simulink model "GolfSwing"  (R2024b)
settings: Solver=VariableStepAuto  StartTime=0.0  StopTime=StopTime  MaxStep=0.001  RelTol=1e-3
PreLoadFcn:
  | cd(matlabdrive);
  | cd '2DModel';
PostLoadFcn:
  | %run SCRIPT_mdlWksGenerate.m;
  | mdlWks=get_param('GolfSwing','ModelWorkspace');
  | mdlWks.DataSource = 'MAT-File';
  | mdlWks.FileName = 'ModelInputs.mat';
  | mdlWks.reload;
model workspace: external: MAT-File ModelInputs.mat (data not in the file)
undefined symbols (not defined in the file or in its folder): GlobalGain, HipConstant, HipDampening, HipTimeGain, KillDampFinalValue, KillDampInitialValue, KillswitchFinalValue, KillswitchInitialValue, KillswitchStepTime, LElbowConstant, LElbowDampening, LElbowTimeGain, LScapConstant, LScapDampening, LScapPositionGain, LScapTimeGain, LShoulderConstant, LShoulderDampening, LShoulderTimeGain, LWristConstant, LWristDampening, LWristTimeGain, RElbowConstant, RElbowDampening, RElbowTimeGain, RScapConstant, RScapDampening, RScapPositionGain, RScapTimeGain, RShoulderConstant, RShoulderDampening, RShoulderTimeGain, RWristConstant, RWristDampening, RWristTimeGain, TorsoConstant, TorsoDampening, TorsoPositionGain, TorsoTimeGain, WristGain, X, Y, Z
libraries: nesl_utility x207, sm_lib x106, matrix_library x11, simulink_extras x2, simulink x1
(part 4 of 6)

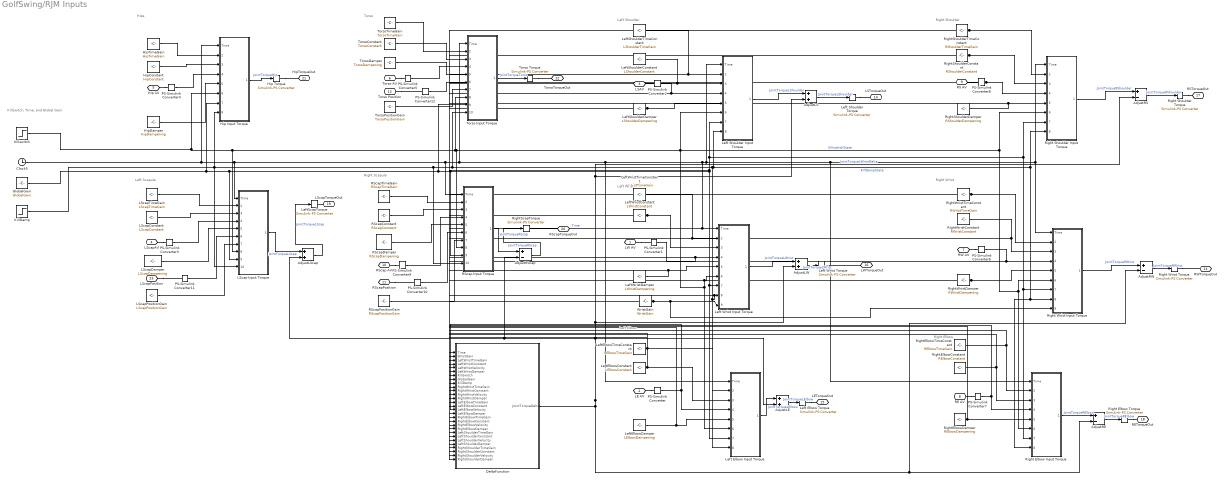
== system GolfSwing/RJM Inputs ==
  note: Killswitch, Time, and Global Gain
  note: Right Scapula
  note: Left Scapula
  note: Left Shoulder
  note: Right Shoulder
  note: Right Elbow
  note: Left Elbow
  note: Torso
  note: Hips
  note: Right Wrist
  note: Left Wrist
  AdjustLE : Sum
  AdjustLS : Sum
  AdjustLScap : Sum
  AdjustLW : Sum
  AdjustRE : Sum  Inputs=+-
  AdjustRS : Sum  Inputs=+-
  AdjustRScap : Sum  Inputs=+-
  AdjustRW : Sum  Inputs=+-
  Clock5 : Clock
  DeltaFunction : MATLAB Function  TreatAsAtomicUnit=on
  GlobalGain : Constant  Value=GlobalGain
  Hip Input Torque : MATLAB Function  TreatAsAtomicUnit=on
  Hip Torque : nesl_utility/Simulink-PS Converter  PhysicalDomain=network_engine_domain  SubClassName=ps_input  LeftPortType=input  RightPortType=output  PseudoPeriodic=off  Frequencies=[]  NoiseDistribution=none  NoiseParameters=[]  Unit=N*m  AffineConversion=off  FilteringAndDerivatives=provide  SimscapeFilterOrder=1  InputFilterTimeConstant=0.001  UdotUserProvided=0
  HipConstant : Constant  Value=HipConstant
  HipDamper : Constant  Value=HipDampening
  HipTimeGain : Constant  Value=HipTimeGain
  KillDamp : Step  Time=KillswitchStepTime  Before=KillDampInitialValue  After=KillDampFinalValue  SampleTime=0
  Killswitch : Step  Time=KillswitchStepTime  Before=KillswitchInitialValue  After=KillswitchFinalValue  SampleTime=0
  LScap Input Torque : MATLAB Function  TreatAsAtomicUnit=on
  LScapConstant : Constant  Value=LScapConstant
  LScapDamper : Constant  Value=LScapDampening
  LScapPositionGain : Constant  Value=LScapPositionGain
  LScapTimeGain : Constant  Value=LScapTimeGain
  Left Elbow Input Torque : MATLAB Function  TreatAsAtomicUnit=on
  Left Elbow Torque : nesl_utility/Simulink-PS Converter  PhysicalDomain=network_engine_domain  SubClassName=ps_input  LeftPortType=input  RightPortType=output  PseudoPeriodic=off  Frequencies=[]  NoiseDistribution=none  NoiseParameters=[]  Unit=N*m  AffineConversion=off  FilteringAndDerivatives=provide  SimscapeFilterOrder=1  InputFilterTimeConstant=0.001  UdotUserProvided=0
  Left Shoulder Input Torque : MATLAB Function  TreatAsAtomicUnit=on
  Left Shoulder Torque : nesl_utility/Simulink-PS Converter  PhysicalDomain=network_engine_domain  SubClassName=ps_input  LeftPortType=input  RightPortType=output  PseudoPeriodic=off  Frequencies=[]  NoiseDistribution=none  NoiseParameters=[]  Unit=N*m  AffineConversion=off  FilteringAndDerivatives=provide  SimscapeFilterOrder=1  InputFilterTimeConstant=0.001  UdotUserProvided=0
  Left Wrist Input Torque : MATLAB Function  TreatAsAtomicUnit=on
  Left Wrist Torque : nesl_utility/Simulink-PS Converter  PhysicalDomain=network_engine_domain  SubClassName=ps_input  LeftPortType=input  RightPortType=output  PseudoPeriodic=off  Frequencies=[]  NoiseDistribution=none  NoiseParameters=[]  Unit=N*m  AffineConversion=off  FilteringAndDerivatives=provide  SimscapeFilterOrder=1  InputFilterTimeConstant=0.001  UdotUserProvided=0
  LeftElbowConstant : Constant  Value=LElbowConstant
  LeftElbowDamper : Constant  Value=LElbowDampening
  LeftElbowTimeConstant : Constant  Value=LElbowTimeGain
  LeftScapTorque : nesl_utility/Simulink-PS Converter  PhysicalDomain=network_engine_domain  SubClassName=ps_input  LeftPortType=input  RightPortType=output  PseudoPeriodic=off  Frequencies=[]  NoiseDistribution=none  NoiseParameters=[]  Unit=N*m  AffineConversion=off  FilteringAndDerivatives=provide  SimscapeFilterOrder=1  InputFilterTimeConstant=0.001  UdotUserProvided=0
  LeftShoulderConstant : Constant  Value=LShoulderConstant
  LeftShoulderDamper : Constant  Value=LShoulderDampening
  LeftShoulderTimeConstant : Constant  Value=LShoulderTimeGain
  LeftWristConstant : Constant  Value=LWristConstant
  LeftWristDamper : Constant  Value=LWristDampening
  LeftWristTimeConstant : Constant  Value=LWristTimeGain
  PS-Simulink Converter{,1..9} (10 alike) : nesl_utility/PS-Simulink Converter  PhysicalDomain=network_engine_domain  SubClassName=ps_output  LeftPortType=input  RightPortType=output  PseudoPeriodic=off  Frequencies=[]  VectorFormat=1-D array  Unit=inherit  AffineConversion=off
  PS-Simulink Converter10 : nesl_utility/PS-Simulink Converter  PhysicalDomain=network_engine_domain  SubClassName=ps_output  LeftPortType=input  RightPortType=output  PseudoPeriodic=off  Frequencies=[]  VectorFormat=inherit  Unit=inherit  AffineConversion=off
  PS-Simulink Converter11 : nesl_utility/PS-Simulink Converter  PhysicalDomain=network_engine_domain  SubClassName=ps_output  LeftPortType=input  RightPortType=output  PseudoPeriodic=off  Frequencies=[]  VectorFormat=inherit  Unit=inherit  AffineConversion=off
  PS-Simulink Converter12 : nesl_utility/PS-Simulink Converter  PhysicalDomain=network_engine_domain  SubClassName=ps_output  LeftPortType=input  RightPortType=output  PseudoPeriodic=off  Frequencies=[]  VectorFormat=inherit  Unit=inherit  AffineConversion=off
  RScap Input Torque : MATLAB Function  TreatAsAtomicUnit=on
  RScapConstant : Constant  Value=RScapConstant
  RScapDamper : Constant  Value=RScapDampening
  RScapPositionGain : Constant  Value=RScapPositionGain
  RScapTimeGain : Constant  Value=RScapTimeGain
  Right Elbow Input Torque : MATLAB Function  TreatAsAtomicUnit=on
  Right Elbow Torque : nesl_utility/Simulink-PS Converter  PhysicalDomain=network_engine_domain  SubClassName=ps_input  LeftPortType=input  RightPortType=output  PseudoPeriodic=off  Frequencies=[]  NoiseDistribution=none  NoiseParameters=[]  Unit=N*m  AffineConversion=off  FilteringAndDerivatives=provide  SimscapeFilterOrder=1  InputFilterTimeConstant=0.001  UdotUserProvided=0
  Right Shoulder Input Torque : MATLAB Function  TreatAsAtomicUnit=on
  Right Shoulder Torque : nesl_utility/Simulink-PS Converter  PhysicalDomain=network_engine_domain  SubClassName=ps_input  LeftPortType=input  RightPortType=output  PseudoPeriodic=off  Frequencies=[]  NoiseDistribution=none  NoiseParameters=[]  Unit=N*m  AffineConversion=off  FilteringAndDerivatives=provide  SimscapeFilterOrder=1  InputFilterTimeConstant=0.001  UdotUserProvided=0
  Right Wrist Input Torque : MATLAB Function  TreatAsAtomicUnit=on
  Right Wrist Torque : nesl_utility/Simulink-PS Converter  PhysicalDomain=network_engine_domain  SubClassName=ps_input  LeftPortType=input  RightPortType=output  PseudoPeriodic=off  Frequencies=[]  NoiseDistribution=none  NoiseParameters=[]  Unit=N*m  AffineConversion=off  FilteringAndDerivatives=provide  SimscapeFilterOrder=1  InputFilterTimeConstant=0.001  UdotUserProvided=0
  RightElbowConstant : Constant  Value=RElbowConstant
  RightElbowDamper : Constant  Value=RElbowDampening
  RightElbowTimeConstant : Constant  Value=RElbowTimeGain
  RightScapTorque : nesl_utility/Simulink-PS Converter  PhysicalDomain=network_engine_domain  SubClassName=ps_input  LeftPortType=input  RightPortType=output  PseudoPeriodic=off  Frequencies=[]  NoiseDistribution=none  NoiseParameters=[]  Unit=N*m  AffineConversion=off  FilteringAndDerivatives=provide  SimscapeFilterOrder=1  InputFilterTimeConstant=0.001  UdotUserProvided=0
  RightShoulderConstant : Constant  Value=RShoulderConstant
  RightShoulderDamper : Constant  Value=RShoulderDampening
  RightShoulderTimeConstant : Constant  Value=RShoulderTimeGain
  RightWristConstant : Constant  Value=RWristConstant
  RightWristDamper : Constant  Value=RWristDampening
  RightWristTimeConstant : Constant  Value=RWristTimeGain
  Torso Input Torque : MATLAB Function  TreatAsAtomicUnit=on
  Torso Torque : nesl_utility/Simulink-PS Converter  PhysicalDomain=network_engine_domain  SubClassName=ps_input  LeftPortType=input  RightPortType=output  PseudoPeriodic=off  Frequencies=[]  NoiseDistribution=none  NoiseParameters=[]  Unit=N*m  AffineConversion=off  FilteringAndDerivatives=provide  SimscapeFilterOrder=1  InputFilterTimeConstant=0.001  UdotUserProvided=0
  TorsoConstant : Constant  Value=TorsoConstant
  TorsoDamper : Constant  Value=TorsoDampening
  TorsoPositionGain : Constant  Value=TorsoPositionGain
  TorsoTimeGain : Constant  Value=TorsoTimeGain
  WristGain : Constant  Value=WristGain
  LW AV : PMIOPort  Side=Left
  LE AV : PMIOPort  Port=2  Side=Left
  LSAV : PMIOPort  Port=3  Side=Left
  LScapAV : PMIOPort  Port=4  Side=Left
  Hip AV : PMIOPort  Port=5  Side=Left
  Torso AV : PMIOPort  Port=6  Side=Left
  RW AV : PMIOPort  Port=7  Side=Left
  RE AV : PMIOPort  Port=8  Side=Left
  RS AV : PMIOPort  Port=9  Side=Left
  RScap AV : PMIOPort  Port=10  Side=Left
  RScapPosition : PMIOPort  Port=11  Side=Left
  Torso Position : PMIOPort  Port=12  Side=Left
  RWTorqueOut : PMIOPort  Port=13  Side=Right
  LSTorqueOut : PMIOPort  Port=14  Side=Right
  LETorqueOut : PMIOPort  Port=15  Side=Right
  LWTorqueOut : PMIOPort  Port=16  Side=Right
  RSTorqueOut : PMIOPort  Port=17  Side=Right
  RETorqueOut : PMIOPort  Port=18  Side=Right
  LScapTorqueOut : PMIOPort  Port=19  Side=Right
  RScapTorqueOut : PMIOPort  Port=20  Side=Right
  HipTorqueOut : PMIOPort  Port=21  Side=Right
  TorsoTorqueOut : PMIOPort  Port=22  Side=Right
  LScapPosition : PMIOPort  Port=23  Side=Right
  wires:
  GlobalGain/1 -> Torso Input Torque/9(GlobalGain), DeltaFunction/8(GlobalGain), Left Shoulder Input Torque/7(GlobalGain), Right Elbow Input Torque/7(GlobalGain), Right Wrist Input Torque/7(GlobalGain), Right Shoulder Input Torque/7(GlobalGain), Left Elbow Input Torque/7(GlobalGain), Left Wrist Input Torque/7(GlobalGain), RScap Input Torque/9(GlobalGain), LScap Input Torque/9(GlobalGain), Hip Input Torque/7(GlobalGain)
  RightElbowConstant/1 -> Right Elbow Input Torque/3(RightElbowConstant), DeltaFunction/19(RightElbowConstant)
  TorsoConstant/1 -> Torso Input Torque/3(TorsoConstant)
  TorsoTimeGain/1 -> Torso Input Torque/2(TorsoTimeGain)
  RightWristConstant/1 -> Right Wrist Input Torque/3(RightWristConstant), DeltaFunction/11(RightWristConstant)
  RightWristTimeConstant/1 -> Right Wrist Input Torque/2(RightWristTimeGain), DeltaFunction/10(RightWristTimeGain)
  RightShoulderConstant/1 -> Right Shoulder Input Torque/3(RightShoulderConstant), DeltaFunction/27(RightShoulderConstant)
  RightShoulderTimeConstant/1 -> Right Shoulder Input Torque/2(RightShoulderTimeGain), DeltaFunction/26(RightShoulderTimeGain)
  RScapConstant/1 -> RScap Input Torque/3(RScapConstant)
  RScapTimeGain/1 -> RScap Input Torque/2(RScapTimeGain)
  HipConstant/1 -> Hip Input Torque/3(HipConstant)
  HipTimeGain/1 -> Hip Input Torque/2(HipTimeGain)
  LeftWristConstant/1 -> Left Wrist Input Torque/3(LeftWristConstant), DeltaFunction/4(LeftWristConstant)
  LeftElbowConstant/1 -> Left Elbow Input Torque/3(LeftElbowConstant), DeltaFunction/15(LeftElbowConstant)
  LeftElbowTimeConstant/1 -> Left Elbow Input Torque/2(LeftElbowTimeGain), DeltaFunction/14(LeftElbowTimeGain)
  LeftShoulderTimeConstant/1 -> DeltaFunction/22(LeftShoulderTimeGain), Left Shoulder Input Torque/2(LeftShoulderTimeGain)
  LeftShoulderConstant/1 -> DeltaFunction/23(LeftShoulderConstant), Left Shoulder Input Torque/3(LeftShoulderConstant)
  LScapTimeGain/1 -> LScap Input Torque/2(LScapTimeGain)
  LScapConstant/1 -> LScap Input Torque/3(LScapConstant)
  TorsoDamper/1 -> Torso Input Torque/5(TorsoDamper)
  HipDamper/1 -> Hip Input Torque/5(HipDamper)
  RightWristDamper/1 -> Right Wrist Input Torque/5(RightWristDamper), DeltaFunction/13(RightWristDamper)
  RightElbowDamper/1 -> Right Elbow Input Torque/5(RightElbowDamper), DeltaFunction/21(RightElbowDamper)
  RightShoulderDamper/1 -> DeltaFunction/29(RightShoulderDamper), Right Shoulder Input Torque/5(RightShoulderDamper)
  RScapDamper/1 -> RScap Input Torque/5(RScapDamper)
  LeftShoulderDamper/1 -> Left Shoulder Input Torque/5(LeftShoulderDamper), DeltaFunction/25(LeftShoulderDamper)
  LScapDamper/1 -> LScap Input Torque/5(LScapDamper)
  LeftElbowDamper/1 -> Left Elbow Input Torque/5(LeftElbowDamper), DeltaFunction/17(LeftElbowDamper)
  LeftWristDamper/1 -> Left Wrist Input Torque/5(LeftWristDamper), DeltaFunction/6(LeftWristDamper)
  PS-Simulink Converter/1 -> Left Elbow Input Torque/4(LeftElbowVelocity), DeltaFunction/16(LeftElbowVelocity)
  PS-Simulink Converter9/1 -> RScap Input Torque/4(RScapVelocity)
  PS-Simulink Converter8/1 -> Right Shoulder Input Torque/4(RightShoulderVelocity), DeltaFunction/28(RightShoulderVelocity)
  PS-Simulink Converter7/1 -> Right Elbow Input Torque/4(RightElbowVelocity), DeltaFunction/20(RightElbowVelocity)
  PS-Simulink Converter6/1 -> DeltaFunction/12(RightWristVelocity), Right Wrist Input Torque/4(RightWristVelocity)
  PS-Simulink Converter5/1 -> Torso Input Torque/4(TorsoVelocity)
  PS-Simulink Converter4/1 -> Hip Input Torque/4(HipVelocity)
  PS-Simulink Converter1/1 -> Left Wrist Input Torque/4(LeftWristVelocity), DeltaFunction/5(LeftWristVelocity)
  PS-Simulink Converter2/1 -> DeltaFunction/24(LeftShoulderVelocity), Left Shoulder Input Torque/4(LeftShoulderVelocity)
  PS-Simulink Converter3/1 -> LScap Input Torque/4(LScapVelocity)
  LScapPositionGain/1 -> LScap Input Torque/7(LScapPositionGain)
  PS-Simulink Converter11/1 -> LScap Input Torque/6(LScapPosition)
  PS-Simulink Converter10/1 -> RScap Input Torque/6(RScapPosition)
  RScapPositionGain/1 -> RScap Input Torque/7(RScapPositionGain)
  TorsoPositionGain/1 -> Torso Input Torque/7(TorsoPositionGain)
  PS-Simulink Converter12/1 -> Torso Input Torque/6(TorsoPosition)
  Hip Input Torque/1(JointTorqueHips) -> Hip Torque/1  "JointTorqueHip"
  Torso Input Torque/1(JointTorqueTorso) -> Torso Torque/1  "JointTorqueTorso"
  Clock5/1 -> Right Wrist Input Torque/1(Time), Right Shoulder Input Torque/1(Time), Right Elbow Input Torque/1(Time), Left Shoulder Input Torque/1(Time), DeltaFunction/1(Time), Left Wrist Input Torque/1(Time), Left Elbow Input Torque/1(Time), Torso Input Torque/1(Time), RScap Input Torque/1(Time), LScap Input Torque/1(Time), Hip Input Torque/1(Time)  "Time"
  Killswitch/1 -> Left Elbow Input Torque/6(Killswitch), Left Wrist Input Torque/6(Killswitch), DeltaFunction/7(Killswitch), Right Wrist Input Torque/6(Killswitch), Right Elbow Input Torque/6(Killswitch), Right Shoulder Input Torque/6(Killswitch), Left Shoulder Input Torque/6(Killswitch), RScap Input Torque/8(Killswitch), Torso Input Torque/8(Killswitch), LScap Input Torque/8(Killswitch), Hip Input Torque/6(Killswitch)  "KillswitchState"
  KillDamp/1 -> Right Elbow Input Torque/8(KillDamp), Right Wrist Input Torque/8(KillDamp), Right Shoulder Input Torque/8(KillDamp), Left Shoulder Input Torque/8(KillDamp), Left Elbow Input Torque/8(KillDamp), DeltaFunction/9(KillDamp), Left Wrist Input Torque/8(KillDamp), Torso Input Torque/10(KillDamp), RScap Input Torque/10(KillDamp), Hip Input Torque/8(KillDamp), LScap Input Torque/10(KillDamp)  "KillDampState"
  Left Elbow Input Torque/1(JointTorqueLElbow) -> AdjustLE/1  "JointTorqueLElbow"
  AdjustLE/1 -> Left Elbow Torque/1  "JointTorqueLElbow"
  AdjustLS/1 -> Left Shoulder Torque/1  "JointTorqueLShoulder"
  AdjustLScap/1 -> LeftScapTorque/1  "JointTorqueLScap"
  LScap Input Torque/1(JointTorqueLScap) -> AdjustLScap/1  "JointTorqueLScap"
  AdjustRScap/1 -> RightScapTorque/1  "JointTorqueRScap"
  AdjustRS/1 -> Right Shoulder Torque/1  "JointTorqueRShoulder"
  AdjustRE/1 -> Right Elbow Torque/1  "JointTorqueRElbow"
  Right Elbow Input Torque/1(JointTorqueRElbow) -> AdjustRE/1  "JointTorqueRElbow"
  RScap Input Torque/1(JointTorqueRScap) -> AdjustRScap/1  "JointTorqueRScap"
  AdjustRW/1 -> Right Wrist Torque/1  "JointTorqueRWrist"
  Right Shoulder Input Torque/1(JointTorqueRShoulder) -> AdjustRS/1  "JointTorqueRShoulder"
  Left Shoulder Input Torque/1(JointTorqueLShoulder) -> AdjustLS/1  "JointTorqueLShoulder"
  AdjustLW/1 -> Left Wrist Torque/1  "JointTorqueLWrist"
  Left Wrist Input Torque/1(JointTorqueLWrist) -> AdjustLW/1  "JointTorqueLWrist"
  Right Wrist Input Torque/1(JointTorqueRWrist) -> AdjustRW/1  "JointTorqueRWrist"
  LeftWristTimeConstant/1 -> Left Wrist Input Torque/2(LeftWristTimeGain), DeltaFunction/3(LeftWristTimeGain)
  DeltaFunction/1(JointTorqueDelta) -> AdjustLScap/2, AdjustRScap/2, AdjustLE/2, AdjustRS/2, AdjustLS/2, AdjustLW/2, AdjustRW/2, AdjustRE/2  "JointTorqueLWristDelta"
  WristGain/1 -> Right Wrist Input Torque/9(WristGain), Left Wrist Input Torque/9(WristGain), DeltaFunction/2(WristGain)
  RightElbowTimeConstant/1 -> Right Elbow Input Torque/2(RightElbowTimeGain), DeltaFunction/18(RightElbowTimeGain)
  connections:
  Torso Torque/RConn1 -- TorsoTorqueOut/RConn1
  Right Shoulder Torque/RConn1 -- RSTorqueOut/RConn1
  Left Shoulder Torque/RConn1 -- LSTorqueOut/RConn1
  Right Elbow Torque/RConn1 -- RETorqueOut/RConn1
  LeftScapTorque/RConn1 -- LScapTorqueOut/RConn1
  RightScapTorque/RConn1 -- RScapTorqueOut/RConn1
  LE AV/RConn1 -- PS-Simulink Converter/LConn1
  LW AV/RConn1 -- PS-Simulink Converter1/LConn1
  LSAV/RConn1 -- PS-Simulink Converter2/LConn1
  LScapAV/RConn1 -- PS-Simulink Converter3/LConn1
  Hip AV/RConn1 -- PS-Simulink Converter4/LConn1
  Torso AV/RConn1 -- PS-Simulink Converter5/LConn1
  RW AV/RConn1 -- PS-Simulink Converter6/LConn1
  RE AV/RConn1 -- PS-Simulink Converter7/LConn1
  RS AV/RConn1 -- PS-Simulink Converter8/LConn1
  RScap AV/RConn1 -- PS-Simulink Converter9/LConn1
  LScapPosition/RConn1 -- PS-Simulink Converter11/LConn1
  RScapPosition/RConn1 -- PS-Simulink Converter10/LConn1
  Torso Position/RConn1 -- PS-Simulink Converter12/LConn1
  Hip Torque/RConn1 -- HipTorqueOut/RConn1
  Left Elbow Torque/RConn1 -- LETorqueOut/RConn1
  Left Wrist Torque/RConn1 -- LWTorqueOut/RConn1
  Right Wrist Torque/RConn1 -- RWTorqueOut/RConn1

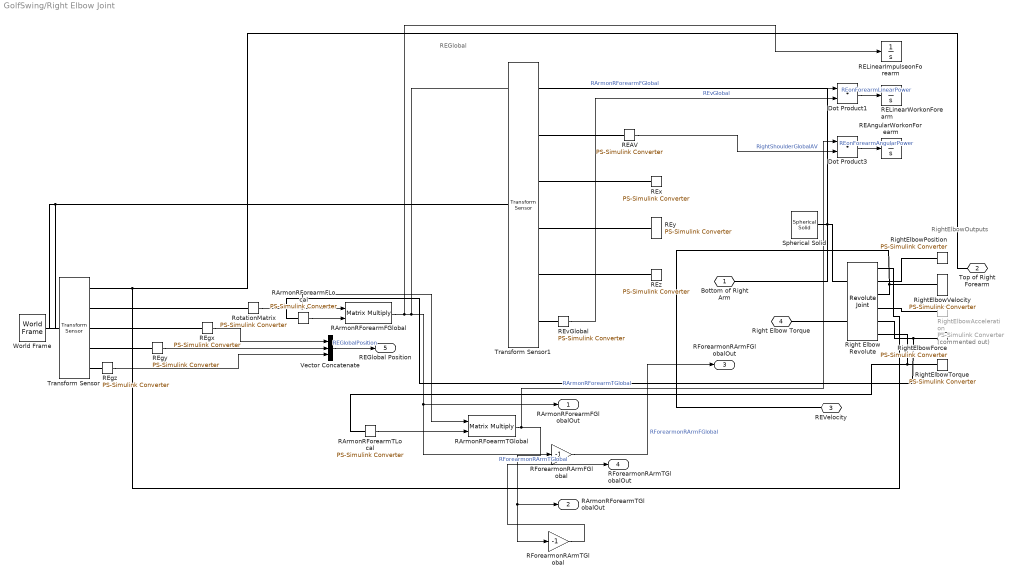
== system GolfSwing/Right Elbow Joint ==
  note: RightElbowOutputs
  note: REGlobal
  Dot Product1 : DotProduct  OutDataTypeStr=Inherit: Inherit via internal rule
  Dot Product3 : DotProduct  OutDataTypeStr=Inherit: Inherit via internal rule
  RArmonRFoearmTGlobal : Product  Multiplication=Matrix(*)
  RArmonRForearmFGlobal : Product  Multiplication=Matrix(*)
  RArmonRForearmFLocal : nesl_utility/PS-Simulink Converter  PhysicalDomain=network_engine_domain  SubClassName=ps_output  LeftPortType=input  RightPortType=output  PseudoPeriodic=off  Frequencies=[]  VectorFormat=1-D array  Unit=inherit  AffineConversion=off
  RArmonRForearmTLocal : nesl_utility/PS-Simulink Converter  PhysicalDomain=network_engine_domain  SubClassName=ps_output  LeftPortType=input  RightPortType=output  PseudoPeriodic=off  Frequencies=[]  VectorFormat=1-D array  Unit=inherit  AffineConversion=off
  REAV : nesl_utility/PS-Simulink Converter  PhysicalDomain=network_engine_domain  SubClassName=ps_output  LeftPortType=input  RightPortType=output  PseudoPeriodic=off  Frequencies=[]  VectorFormat=1-D array  Unit=inherit  AffineConversion=off
  REAngularWorkonForearm : Integrator
  RELinearImpulseonForearm : Integrator
  RELinearWorkonForearm : Integrator
  REgx : nesl_utility/PS-Simulink Converter  PhysicalDomain=network_engine_domain  SubClassName=ps_output  LeftPortType=input  RightPortType=output  PseudoPeriodic=off  Frequencies=[]  VectorFormat=1-D array  Unit=inherit  AffineConversion=off
  REgy : nesl_utility/PS-Simulink Converter  PhysicalDomain=network_engine_domain  SubClassName=ps_output  LeftPortType=input  RightPortType=output  PseudoPeriodic=off  Frequencies=[]  VectorFormat=1-D array  Unit=inherit  AffineConversion=off
  REgz : nesl_utility/PS-Simulink Converter  PhysicalDomain=network_engine_domain  SubClassName=ps_output  LeftPortType=input  RightPortType=output  PseudoPeriodic=off  Frequencies=[]  VectorFormat=1-D array  Unit=inherit  AffineConversion=off
  REvGlobal : nesl_utility/PS-Simulink Converter  PhysicalDomain=network_engine_domain  SubClassName=ps_output  LeftPortType=input  RightPortType=output  PseudoPeriodic=off  Frequencies=[]  VectorFormat=1-D array  Unit=inherit  AffineConversion=off
  REx : nesl_utility/PS-Simulink Converter  PhysicalDomain=network_engine_domain  SubClassName=ps_output  LeftPortType=input  RightPortType=output  PseudoPeriodic=off  Frequencies=[]  VectorFormat=1-D array  Unit=inherit  AffineConversion=off
  REy : nesl_utility/PS-Simulink Converter  PhysicalDomain=network_engine_domain  SubClassName=ps_output  LeftPortType=input  RightPortType=output  PseudoPeriodic=off  Frequencies=[]  VectorFormat=1-D array  Unit=inherit  AffineConversion=off
  REz : nesl_utility/PS-Simulink Converter  PhysicalDomain=network_engine_domain  SubClassName=ps_output  LeftPortType=input  RightPortType=output  PseudoPeriodic=off  Frequencies=[]  VectorFormat=1-D array  Unit=inherit  AffineConversion=off
  RForearmonRArmFGlobal : Gain  Gain=-1
  RForearmonRArmTGlobal : Gain  Gain=-1
  Right Elbow Revolute : sm_lib/Joints/Revolute Joint  JointMode=Normal  CompositeWrenchDir=BaseOnFollower  CompositeWrenchFrame=FollowerFrame  SenseConstraintForce=off  SenseConstraintTorque=off  SenseTotalForce=on  SenseTotalTorque=on  PositionTargetSpecify=off  PositionTargetPriority=Low  PositionTargetValue=75  PositionTargetValueUnits=deg  VelocityTargetSpecify=on  VelocityTargetPriority=High  VelocityTargetValue=RElbowStartVelocity  VelocityTargetValueUnits=deg/s  EquilibriumPosition=0  EquilibriumPositionUnits=deg  SpringStiffness=0  SpringStiffnessUnits=N*m/deg  DampingCoefficient=0  DampingCoefficientUnits=N*m/(deg/s)  LowerLimitSpecify=off  LowerLimitBound=-120  LowerLimitBoundUnits=deg  LowerLimitStiffness=1.5  LowerLimitStiffnessUnits=N*m/deg  LowerLimitDamping=0  LowerLimitDampingUnits=N*m/(deg/s)  LowerLimitTransitionRegionWidth=0.1  LowerLimitTransitionRegionWidthUnits=deg  UpperLimitSpecify=off  UpperLimitBound=0  UpperLimitBoundUnits=deg  UpperLimitStiffness=1  UpperLimitStiffnessUnits=N*m/deg  UpperLimitDamping=0  UpperLimitDampingUnits=N*m/(deg/s)  UpperLimitTransitionRegionWidth=0.1  UpperLimitTransitionRegionWidthUnits=deg  TorqueActuationMode=InputTorque  MotionActuationMode=ComputedMotion  SensePosition=on  SenseVelocity=on  SenseAcceleration=on  SenseTorqueForce=off  SenseLowerLimitTorqueForce=off  SenseUpperLimitTorqueForce=off
      settings: LogSimulationData=on
  RightElbowAcceleration : nesl_utility/PS-Simulink Converter  Commented=on  PhysicalDomain=network_engine_domain  SubClassName=ps_output  LeftPortType=input  RightPortType=output  PseudoPeriodic=off  Frequencies=[]  VectorFormat=1-D array  Unit=inherit  AffineConversion=off
  RightElbowForce : nesl_utility/PS-Simulink Converter  PhysicalDomain=network_engine_domain  SubClassName=ps_output  LeftPortType=input  RightPortType=output  PseudoPeriodic=off  Frequencies=[]  VectorFormat=1-D array  Unit=inherit  AffineConversion=off
  RightElbowPosition : nesl_utility/PS-Simulink Converter  PhysicalDomain=network_engine_domain  SubClassName=ps_output  LeftPortType=input  RightPortType=output  PseudoPeriodic=off  Frequencies=[]  VectorFormat=1-D array  Unit=inherit  AffineConversion=off
  RightElbowTorque : nesl_utility/PS-Simulink Converter  PhysicalDomain=network_engine_domain  SubClassName=ps_output  LeftPortType=input  RightPortType=output  PseudoPeriodic=off  Frequencies=[]  VectorFormat=1-D array  Unit=inherit  AffineConversion=off
  RightElbowVelocity : nesl_utility/PS-Simulink Converter  PhysicalDomain=network_engine_domain  SubClassName=ps_output  LeftPortType=input  RightPortType=output  PseudoPeriodic=off  Frequencies=[]  VectorFormat=1-D array  Unit=inherit  AffineConversion=off
  RotationMatrix : nesl_utility/PS-Simulink Converter  PhysicalDomain=network_engine_domain  SubClassName=ps_output  LeftPortType=input  RightPortType=output  PseudoPeriodic=off  Frequencies=[]  VectorFormat=1-D array  Unit=inherit  AffineConversion=off
  Spherical Solid : sm_lib/Body Elements/Spherical Solid  SphereRadius=1.75  SphereRadiusUnits=in  ExportEntireGeometry=off  InertiaType=CalculateFromGeometry  BasedOnType=Density  Density=0  DensityUnits=kg/m^3  Mass=1  MassUnits=kg  CenterOfMass=[0 0 0]  CenterOfMassUnits=m  MomentsOfInertia=[1 1 1]  MomentsOfInertiaUnits=kg*m^2  ProductsOfInertia=[0 0 0]  ProductsOfInertiaUnits=kg*m^2  GraphicType=FromGeometry  MarkerShape=Sphere  MarkerSize=10  GraphicVisPropType=SimpleVisualProperties  GraphicDiffuseColor=[1.0 0.8 0.4]  GraphicOpacity=1  GraphicSpecularColor=[0.5 0.5 0.5 1.0]  GraphicAmbientColor=[0.15 0.15 0.15 1.0]  GraphicEmissiveColor=[0.0 0.0 0.0 1.0]  GraphicShininess=75  DoExposeReferenceFrame=on  SerializedFrames=<Frames/>
  Transform Sensor : sm_lib/Frames and Transforms/Transform Sensor  MeasurementFrame=World  RotationSequence=XYX  SenseAngle=off  SenseAxis=off  SenseQ=off  SenseR=on  SenseRotationSequence=off  SenseOmegaX=off  SenseOmegaY=off  SenseOmegaZ=off  SenseOmega=off  SenseQDot=off  SenseRDot=off  SenseRotationSequenceDot=off  SenseAlphaX=off  SenseAlphaY=off  SenseAlphaZ=off  SenseAlpha=off  SenseQDDot=off  SenseRDDot=off  SenseX=on  SenseY=on  SenseZ=on  SenseXYZ=off  SenseRad=off  SenseAzim=off  SenseDist=off  SenseInc=off  SenseXDot=off  SenseYDot=off  SenseZDot=off  SenseXYZDot=off  SenseRadDot=off  SenseAzimDot=off  SenseDistDot=off  SenseIncDot=off  SenseXDDot=off  SenseYDDot=off  SenseZDDot=off  SenseXYZDDot=off  SenseRadDDot=off  SenseAzimDDot=off  SenseDistDDot=off  SenseIncDDot=off
  Transform Sensor1 : sm_lib/Frames and Transforms/Transform Sensor  MeasurementFrame=World  RotationSequence=XYX  SenseAngle=off  SenseAxis=off  SenseQ=off  SenseR=off  SenseRotationSequence=off  SenseOmegaX=off  SenseOmegaY=off  SenseOmegaZ=off  SenseOmega=on  SenseQDot=off  SenseRDot=off  SenseRotationSequenceDot=off  SenseAlphaX=off  SenseAlphaY=off  SenseAlphaZ=off  SenseAlpha=off  SenseQDDot=off  SenseRDDot=off  SenseX=on  SenseY=on  SenseZ=on  SenseXYZ=off  SenseRad=off  SenseAzim=off  SenseDist=off  SenseInc=off  SenseXDot=off  SenseYDot=off  SenseZDot=off  SenseXYZDot=on  SenseRadDot=off  SenseAzimDot=off  SenseDistDot=off  SenseIncDot=off  SenseXDDot=off  SenseYDDot=off  SenseZDDot=off  SenseXYZDDot=off  SenseRadDDot=off  SenseAzimDDot=off  SenseDistDDot=off  SenseIncDDot=off
  Vector Concatenate : Concatenate  NumInputs=3
  World Frame : sm_lib/Frames and Transforms/World Frame
  Bottom of Right Arm : PMIOPort  Side=Left
  Top of Right Forearm : PMIOPort  Port=2  Side=Right
  REVelocity : PMIOPort  Port=3  Side=Right
  Right Elbow Torque : PMIOPort  Port=4  Side=Right
  RArmonRForearmFGlobalOut : Outport
  RArmonRForearmTGlobalOut : Outport  Port=2
  RForearmonRArmFGlobalOut : Outport  Port=3
  RForearmonRArmTGlobalOut : Outport  Port=4
  REGlobal Position : Outport  Port=5
  wires:
  RArmonRForearmFLocal/1 -> RArmonRForearmFGlobal/2
  RotationMatrix/1 -> RArmonRForearmFGlobal/1, RArmonRFoearmTGlobal/1
  RArmonRForearmTLocal/1 -> RArmonRFoearmTGlobal/2
  RForearmonRArmTGlobal/1 -> RForearmonRArmTGlobalOut/1  "RForearmonRArmTGlobal"
  RArmonRForearmFGlobal/1 -> RArmonRForearmFGlobalOut/1, RForearmonRArmFGlobal/1, Dot Product1/1, RELinearImpulseonForearm/1  "RArmonRForearmFGlobal"
  RForearmonRArmFGlobal/1 -> RForearmonRArmFGlobalOut/1  "RForearmonRArmFGlobal"
  RArmonRFoearmTGlobal/1 -> RArmonRForearmTGlobalOut/1, RForearmonRArmTGlobal/1, Dot Product3/1  "RArmonRForearmTGlobal"
  REgx/1 -> Vector Concatenate/1
  REgz/1 -> Vector Concatenate/3
  Vector Concatenate/1 -> REGlobal Position/1  "REGlobalPosition"
  REgy/1 -> Vector Concatenate/2
  Dot Product3/1 -> REAngularWorkonForearm/1  "REonForearmAngularPower"
  Dot Product1/1 -> RELinearWorkonForearm/1  "REonForearmLinearPower"
  REvGlobal/1 -> Dot Product1/2  "REvGlobal"
  REAV/1 -> Dot Product3/2  "RightShoulderGlobalAV"
  connections:
  Top of Right Forearm/RConn1 -- Transform Sensor/RConn1 -- Right Elbow Revolute/RConn1
  Bottom of Right Arm/RConn1 -- Right Elbow Revolute/LConn1 -- Transform Sensor1/RConn1 -- Spherical Solid/RConn1
  Right Elbow Torque/RConn1 -- Right Elbow Revolute/LConn2
  REgx/LConn1 -- Transform Sensor/RConn3
  REgy/LConn1 -- Transform Sensor/RConn4
  World Frame/RConn1 -- Transform Sensor1/LConn1 -- Transform Sensor/LConn1
  Transform Sensor/RConn5 -- REgz/LConn1
  RotationMatrix/LConn1 -- Transform Sensor/RConn2
  REvGlobal/LConn1 -- Transform Sensor1/RConn6
  REAV/LConn1 -- Transform Sensor1/RConn2
  REz/LConn1 -- Transform Sensor1/RConn5
  REy/LConn1 -- Transform Sensor1/RConn4
  REx/LConn1 -- Transform Sensor1/RConn3
  Right Elbow Revolute/RConn2 -- RightElbowPosition/LConn1
  Right Elbow Revolute/RConn3 -- RightElbowVelocity/LConn1 -- REVelocity/RConn1
  Right Elbow Revolute/RConn5 -- RightElbowForce/LConn1 -- RArmonRForearmFLocal/LConn1
  Right Elbow Revolute/RConn6 -- RightElbowTorque/LConn1 -- RArmonRForearmTLocal/LConn1
  Right Elbow Revolute/RConn4 -- RightElbowAcceleration/LConn1

== system GolfSwing/Right Forearm MOF ==
  RW Global Position In : Inport
  RE Global Position : Inport  Port=2
  RArmonRForearmFGlobalIn : Inport  Port=3
  RArmonRForearmTGlobalIn : Inport  Port=4
  RWristonRForearmFGlobalIn : Inport  Port=5
  RWristonRForearmTGlobalIn : Inport  Port=6
  R Vector Elbow Force on Right Forearm : Sum  Inputs=-+
  R Vector Wrist Force on Right Forearm : Sum  Inputs=-+
  RArmonRForearmMOFGlobal : matrix_library/Cross Product
  REAngularImpulseonForearm : Integrator
  RElbowonRForearmMOFLocal : Product  Multiplication=Matrix(*)
  RFCOM : sm_lib/Body Elements/Inertia Sensor  SensorExtent=BodyGroup  SpanWeldJoints=off  ExcludeGroundedBodies=off  MeasurementFrame=World  SenseMass=off  SenseCenterOfMass=on  SenseInertiaMatrix=off  SenseCenteredInertiaMatrix=off  SensePrincipalInertiaMatrix=off  SenseRotationMatrix=off  GraphicType=None  PrincipalInertiaFrameSize=20  GraphicVisPropType=SimpleVisualProperties  GraphicDiffuseColor=[0.5 0.5 0.5]  GraphicOpacity=1  GraphicSpecularColor=[0.5 0.5 0.5 1.0]  GraphicAmbientColor=[0.15 0.15 0.15 1.0]  GraphicEmissiveColor=[0.0 0.0 0.0 1.0]  GraphicShininess=75
  RWristonRForearmMOFGlobal : matrix_library/Cross Product
  RWristonRForearmMOFLocal : Product  Multiplication=Matrix(*)
  Right Forearm COM : nesl_utility/PS-Simulink Converter  PhysicalDomain=network_engine_domain  SubClassName=ps_output  LeftPortType=input  RightPortType=output  PseudoPeriodic=off  Frequencies=[]  VectorFormat=1-D array  Unit=inherit  AffineConversion=off
  RotationTransformRightForearm : nesl_utility/PS-Simulink Converter  PhysicalDomain=network_engine_domain  SubClassName=ps_output  LeftPortType=input  RightPortType=output  PseudoPeriodic=off  Frequencies=[]  VectorFormat=1-D array  Unit=inherit  AffineConversion=off
  SumofMomentsLeftArmGlobal : Sum  Inputs=++++
  SumofMomentsREonRForearm : Sum
  SumofMomentsRForearmLocal : Product  Multiplication=Matrix(*)
  Transform Sensor : sm_lib/Frames and Transforms/Transform Sensor  MeasurementFrame=World  RotationSequence=XYX  SenseAngle=off  SenseAxis=off  SenseQ=off  SenseR=on  SenseRotationSequence=off  SenseOmegaX=off  SenseOmegaY=off  SenseOmegaZ=off  SenseOmega=off  SenseQDot=off  SenseRDot=off  SenseRotationSequenceDot=off  SenseAlphaX=off  SenseAlphaY=off  SenseAlphaZ=off  SenseAlpha=off  SenseQDDot=off  SenseRDDot=off  SenseX=off  SenseY=off  SenseZ=off  SenseXYZ=off  SenseRad=off  SenseAzim=off  SenseDist=off  SenseInc=off  SenseXDot=off  SenseYDot=off  SenseZDot=off  SenseXYZDot=off  SenseRadDot=off  SenseAzimDot=off  SenseDistDot=off  SenseIncDot=off  SenseXDDot=off  SenseYDDot=off  SenseZDDot=off  SenseXYZDDot=off  SenseRadDDot=off  SenseAzimDDot=off  SenseDistDDot=off  SenseIncDDot=off
  World Frame : sm_lib/Frames and Transforms/World Frame
  Right Forearm : PMIOPort  Side=Left
  wires:
  Right Forearm COM/1 -> R Vector Elbow Force on Right Forearm/1, R Vector Wrist Force on Right Forearm/1  "RightForearmCOM"
  RW Global Position In/1 -> R Vector Wrist Force on Right Forearm/2
  RE Global Position/1 -> R Vector Elbow Force on Right Forearm/2
  R Vector Elbow Force on Right Forearm/1 -> RArmonRForearmMOFGlobal/1
  RArmonRForearmFGlobalIn/1 -> RArmonRForearmMOFGlobal/2
  R Vector Wrist Force on Right Forearm/1 -> RWristonRForearmMOFGlobal/1
  RWristonRForearmTGlobalIn/1 -> SumofMomentsLeftArmGlobal/4
  RWristonRForearmFGlobalIn/1 -> RWristonRForearmMOFGlobal/2
  SumofMomentsLeftArmGlobal/1 -> SumofMomentsRForearmLocal/2  "SumonMomentsLeftArmGlobal"
  RWristonRForearmMOFGlobal/1 -> RWristonRForearmMOFLocal/2, SumofMomentsLeftArmGlobal/2  "RWristonRForearmMOFGlobal"
  RotationTransformRightForearm/1 -> SumofMomentsRForearmLocal/1, RWristonRForearmMOFLocal/1, RElbowonRForearmMOFLocal/1
  SumofMomentsREonRForearm/1 -> REAngularImpulseonForearm/1  "SumofMomentsREonRForearm"
  RArmonRForearmTGlobalIn/1 -> SumofMomentsLeftArmGlobal/3, SumofMomentsREonRForearm/1
  RArmonRForearmMOFGlobal/1 -> SumofMomentsREonRForearm/2, RElbowonRForearmMOFLocal/2, SumofMomentsLeftArmGlobal/1  "RElbowonRForearmMOFGlobal"
  connections:
  Right Forearm COM/LConn1 -- RFCOM/RConn1
  RFCOM/LConn1 -- Right Forearm/RConn1 -- Transform Sensor/LConn1
  Transform Sensor/RConn1 -- World Frame/RConn1
  RotationTransformRightForearm/LConn1 -- Transform Sensor/RConn2

== system GolfSwing/Right Scapula Joint ==
  note: RSOutput
  RScapForce : nesl_utility/PS-Simulink Converter  PhysicalDomain=network_engine_domain  SubClassName=ps_output  LeftPortType=input  RightPortType=output  PseudoPeriodic=off  Frequencies=[]  VectorFormat=1-D array  Unit=inherit  AffineConversion=off
  RScapPosition : nesl_utility/PS-Simulink Converter  PhysicalDomain=network_engine_domain  SubClassName=ps_output  LeftPortType=input  RightPortType=output  PseudoPeriodic=off  Frequencies=[]  VectorFormat=1-D array  Unit=inherit  AffineConversion=off
  RScapTorque1 : nesl_utility/PS-Simulink Converter  PhysicalDomain=network_engine_domain  SubClassName=ps_output  LeftPortType=input  RightPortType=output  PseudoPeriodic=off  Frequencies=[]  VectorFormat=1-D array  Unit=inherit  AffineConversion=off
  RScapVel : nesl_utility/PS-Simulink Converter  PhysicalDomain=network_engine_domain  SubClassName=ps_output  LeftPortType=input  RightPortType=output  PseudoPeriodic=off  Frequencies=[]  VectorFormat=1-D array  Unit=inherit  AffineConversion=off
  Right Scapula : sm_lib/Joints/Revolute Joint  JointMode=Normal  CompositeWrenchDir=BaseOnFollower  CompositeWrenchFrame=FollowerFrame  SenseConstraintForce=off  SenseConstraintTorque=off  SenseTotalForce=on  SenseTotalTorque=on  PositionTargetSpecify=on  PositionTargetPriority=High  PositionTargetValue=RScapStartPosition  PositionTargetValueUnits=deg  VelocityTargetSpecify=on  VelocityTargetPriority=High  VelocityTargetValue=RScapStartVelocity  VelocityTargetValueUnits=deg/s  EquilibriumPosition=0  EquilibriumPositionUnits=deg  SpringStiffness=0  SpringStiffnessUnits=N*m/deg  DampingCoefficient=0  DampingCoefficientUnits=N*m/(deg/s)  LowerLimitSpecify=off  LowerLimitBound=-90  LowerLimitBoundUnits=deg  LowerLimitStiffness=1e4  LowerLimitStiffnessUnits=N*m/deg  LowerLimitDamping=10  LowerLimitDampingUnits=N*m/(deg/s)  LowerLimitTransitionRegionWidth=0.1  LowerLimitTransitionRegionWidthUnits=deg  UpperLimitSpecify=off  UpperLimitBound=90  UpperLimitBoundUnits=deg  UpperLimitStiffness=1e4  UpperLimitStiffnessUnits=N*m/deg  UpperLimitDamping=10  UpperLimitDampingUnits=N*m/(deg/s)  UpperLimitTransitionRegionWidth=0.1  UpperLimitTransitionRegionWidthUnits=deg  TorqueActuationMode=InputTorque  MotionActuationMode=ComputedMotion  SensePosition=on  SenseVelocity=on  SenseAcceleration=off  SenseTorqueForce=off  SenseLowerLimitTorqueForce=off  SenseUpperLimitTorqueForce=off
  RScapTorque : PMIOPort  Side=Left
  COMRodTop : PMIOPort  Port=2  Side=Left
  RSV : PMIOPort  Port=3  Side=Left
  RSP : PMIOPort  Port=4  Side=Left
  Hub : PMIOPort  Port=5  Side=Right
  connections:
  Right Scapula/LConn2 -- RScapTorque/RConn1
  Right Scapula/RConn2 -- RScapPosition/LConn1 -- RSP/RConn1
  Right Scapula/LConn1 -- COMRodTop/RConn1
  Hub/RConn1 -- Right Scapula/RConn1
  Right Scapula/RConn4 -- RScapForce/LConn1
  Right Scapula/RConn5 -- RScapTorque1/LConn1
  RSV/RConn1 -- Right Scapula/RConn3 -- RScapVel/LConn1

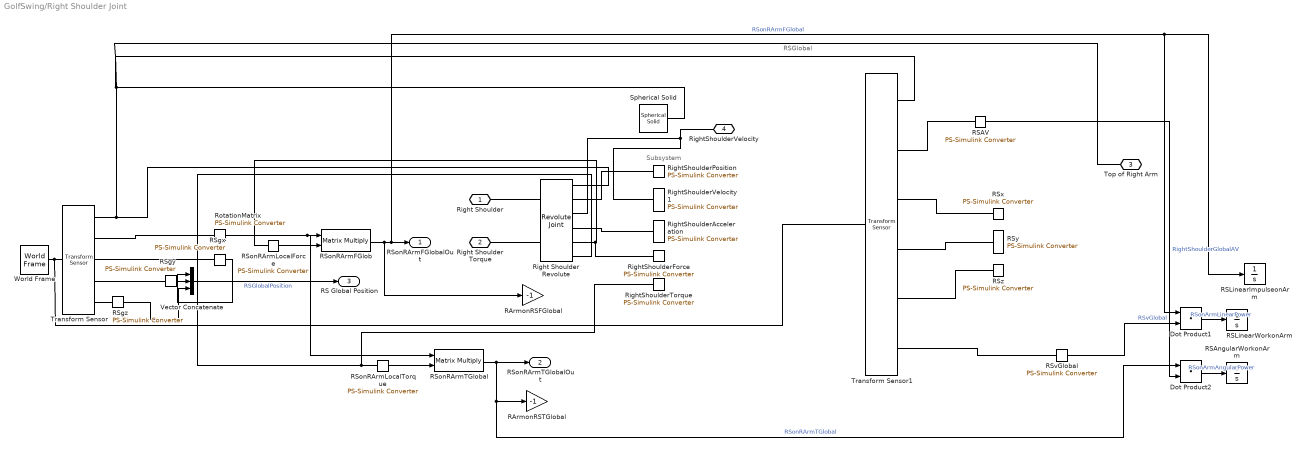
== system GolfSwing/Right Shoulder Joint ==
  note: RSGlobal
  note: Subsystem
  Dot Product1 : DotProduct  OutDataTypeStr=Inherit: Inherit via internal rule
  Dot Product2 : DotProduct  OutDataTypeStr=Inherit: Inherit via internal rule
  RArmonRSFGlobal : Gain  Gain=-1
  RArmonRSTGlobal : Gain  Gain=-1
  RSAV : nesl_utility/PS-Simulink Converter  PhysicalDomain=network_engine_domain  SubClassName=ps_output  LeftPortType=input  RightPortType=output  PseudoPeriodic=off  Frequencies=[]  VectorFormat=1-D array  Unit=inherit  AffineConversion=off
  RSAngularWorkonArm : Integrator
  RSLinearImpulseonArm : Integrator
  RSLinearWorkonArm : Integrator
  RSgx : nesl_utility/PS-Simulink Converter  PhysicalDomain=network_engine_domain  SubClassName=ps_output  LeftPortType=input  RightPortType=output  PseudoPeriodic=off  Frequencies=[]  VectorFormat=1-D array  Unit=inherit  AffineConversion=off
  RSgy : nesl_utility/PS-Simulink Converter  PhysicalDomain=network_engine_domain  SubClassName=ps_output  LeftPortType=input  RightPortType=output  PseudoPeriodic=off  Frequencies=[]  VectorFormat=1-D array  Unit=inherit  AffineConversion=off
  RSgz : nesl_utility/PS-Simulink Converter  PhysicalDomain=network_engine_domain  SubClassName=ps_output  LeftPortType=input  RightPortType=output  PseudoPeriodic=off  Frequencies=[]  VectorFormat=1-D array  Unit=inherit  AffineConversion=off
  RSonRArmFGlob : Product  Multiplication=Matrix(*)
  RSonRArmLocalForce : nesl_utility/PS-Simulink Converter  PhysicalDomain=network_engine_domain  SubClassName=ps_output  LeftPortType=input  RightPortType=output  PseudoPeriodic=off  Frequencies=[]  VectorFormat=1-D array  Unit=inherit  AffineConversion=off
  RSonRArmLocalTorque : nesl_utility/PS-Simulink Converter  PhysicalDomain=network_engine_domain  SubClassName=ps_output  LeftPortType=input  RightPortType=output  PseudoPeriodic=off  Frequencies=[]  VectorFormat=1-D array  Unit=inherit  AffineConversion=off
  RSonRArmTGlobal : Product  Multiplication=Matrix(*)
  RSvGlobal : nesl_utility/PS-Simulink Converter  PhysicalDomain=network_engine_domain  SubClassName=ps_output  LeftPortType=input  RightPortType=output  PseudoPeriodic=off  Frequencies=[]  VectorFormat=1-D array  Unit=inherit  AffineConversion=off
  RSx : nesl_utility/PS-Simulink Converter  PhysicalDomain=network_engine_domain  SubClassName=ps_output  LeftPortType=input  RightPortType=output  PseudoPeriodic=off  Frequencies=[]  VectorFormat=1-D array  Unit=inherit  AffineConversion=off
  RSy : nesl_utility/PS-Simulink Converter  PhysicalDomain=network_engine_domain  SubClassName=ps_output  LeftPortType=input  RightPortType=output  PseudoPeriodic=off  Frequencies=[]  VectorFormat=1-D array  Unit=inherit  AffineConversion=off
  RSz : nesl_utility/PS-Simulink Converter  PhysicalDomain=network_engine_domain  SubClassName=ps_output  LeftPortType=input  RightPortType=output  PseudoPeriodic=off  Frequencies=[]  VectorFormat=1-D array  Unit=inherit  AffineConversion=off
  Right Shoulder Revolute : sm_lib/Joints/Revolute Joint  JointMode=Normal  CompositeWrenchDir=BaseOnFollower  CompositeWrenchFrame=FollowerFrame  SenseConstraintForce=off  SenseConstraintTorque=off  SenseTotalForce=on  SenseTotalTorque=on  PositionTargetSpecify=on  PositionTargetPriority=Low  PositionTargetValue=RShoulderStartPosition  PositionTargetValueUnits=deg  VelocityTargetSpecify=on  VelocityTargetPriority=High  VelocityTargetValue=RShoulderStartVelocity  VelocityTargetValueUnits=deg/s  EquilibriumPosition=0  EquilibriumPositionUnits=deg  SpringStiffness=0  SpringStiffnessUnits=N*m/deg  DampingCoefficient=0  DampingCoefficientUnits=N*m/(deg/s)  LowerLimitSpecify=off  LowerLimitBound=-150  LowerLimitBoundUnits=deg  LowerLimitStiffness=1e4  LowerLimitStiffnessUnits=N*m/deg  LowerLimitDamping=10  LowerLimitDampingUnits=N*m/(deg/s)  LowerLimitTransitionRegionWidth=0.1  LowerLimitTransitionRegionWidthUnits=deg  UpperLimitSpecify=off  UpperLimitBound=65  UpperLimitBoundUnits=deg  UpperLimitStiffness=1e4  UpperLimitStiffnessUnits=N*m/deg  UpperLimitDamping=10  UpperLimitDampingUnits=N*m/(deg/s)  UpperLimitTransitionRegionWidth=0.1  UpperLimitTransitionRegionWidthUnits=deg  TorqueActuationMode=InputTorque  MotionActuationMode=ComputedMotion  SensePosition=on  SenseVelocity=on  SenseAcceleration=on  SenseTorqueForce=off  SenseLowerLimitTorqueForce=off  SenseUpperLimitTorqueForce=off
      settings: LogSimulationData=on
  RightShoulderAcceleration : nesl_utility/PS-Simulink Converter  PhysicalDomain=network_engine_domain  SubClassName=ps_output  LeftPortType=input  RightPortType=output  PseudoPeriodic=off  Frequencies=[]  VectorFormat=1-D array  Unit=inherit  AffineConversion=off
  RightShoulderForce : nesl_utility/PS-Simulink Converter  PhysicalDomain=network_engine_domain  SubClassName=ps_output  LeftPortType=input  RightPortType=output  PseudoPeriodic=off  Frequencies=[]  VectorFormat=1-D array  Unit=inherit  AffineConversion=off
  RightShoulderPosition : nesl_utility/PS-Simulink Converter  PhysicalDomain=network_engine_domain  SubClassName=ps_output  LeftPortType=input  RightPortType=output  PseudoPeriodic=off  Frequencies=[]  VectorFormat=1-D array  Unit=inherit  AffineConversion=off
  RightShoulderTorque : nesl_utility/PS-Simulink Converter  PhysicalDomain=network_engine_domain  SubClassName=ps_output  LeftPortType=input  RightPortType=output  PseudoPeriodic=off  Frequencies=[]  VectorFormat=1-D array  Unit=inherit  AffineConversion=off
  RightShoulderVelocity1 : nesl_utility/PS-Simulink Converter  PhysicalDomain=network_engine_domain  SubClassName=ps_output  LeftPortType=input  RightPortType=output  PseudoPeriodic=off  Frequencies=[]  VectorFormat=1-D array  Unit=inherit  AffineConversion=off
  RotationMatrix : nesl_utility/PS-Simulink Converter  PhysicalDomain=network_engine_domain  SubClassName=ps_output  LeftPortType=input  RightPortType=output  PseudoPeriodic=off  Frequencies=[]  VectorFormat=1-D array  Unit=inherit  AffineConversion=off
  Spherical Solid : sm_lib/Body Elements/Spherical Solid  SphereRadius=1.75  SphereRadiusUnits=in  ExportEntireGeometry=off  InertiaType=CalculateFromGeometry  BasedOnType=Density  Density=0  DensityUnits=kg/m^3  Mass=1  MassUnits=kg  CenterOfMass=[0 0 0]  CenterOfMassUnits=m  MomentsOfInertia=[1 1 1]  MomentsOfInertiaUnits=kg*m^2  ProductsOfInertia=[0 0 0]  ProductsOfInertiaUnits=kg*m^2  GraphicType=FromGeometry  MarkerShape=Sphere  MarkerSize=10  GraphicVisPropType=SimpleVisualProperties  GraphicDiffuseColor=[0.2 0.2 1.0]  GraphicOpacity=1  GraphicSpecularColor=[0.5 0.5 0.5 1.0]  GraphicAmbientColor=[0.15 0.15 0.15 1.0]  GraphicEmissiveColor=[0.0 0.0 0.0 1.0]  GraphicShininess=75  DoExposeReferenceFrame=on  SerializedFrames=<Frames/>
  Transform Sensor : sm_lib/Frames and Transforms/Transform Sensor  MeasurementFrame=World  RotationSequence=XYX  SenseAngle=off  SenseAxis=off  SenseQ=off  SenseR=on  SenseRotationSequence=off  SenseOmegaX=off  SenseOmegaY=off  SenseOmegaZ=off  SenseOmega=off  SenseQDot=off  SenseRDot=off  SenseRotationSequenceDot=off  SenseAlphaX=off  SenseAlphaY=off  SenseAlphaZ=off  SenseAlpha=off  SenseQDDot=off  SenseRDDot=off  SenseX=on  SenseY=on  SenseZ=on  SenseXYZ=off  SenseRad=off  SenseAzim=off  SenseDist=off  SenseInc=off  SenseXDot=off  SenseYDot=off  SenseZDot=off  SenseXYZDot=off  SenseRadDot=off  SenseAzimDot=off  SenseDistDot=off  SenseIncDot=off  SenseXDDot=off  SenseYDDot=off  SenseZDDot=off  SenseXYZDDot=off  SenseRadDDot=off  SenseAzimDDot=off  SenseDistDDot=off  SenseIncDDot=off
  Transform Sensor1 : sm_lib/Frames and Transforms/Transform Sensor  MeasurementFrame=World  RotationSequence=XYX  SenseAngle=off  SenseAxis=off  SenseQ=off  SenseR=off  SenseRotationSequence=off  SenseOmegaX=off  SenseOmegaY=off  SenseOmegaZ=off  SenseOmega=on  SenseQDot=off  SenseRDot=off  SenseRotationSequenceDot=off  SenseAlphaX=off  SenseAlphaY=off  SenseAlphaZ=off  SenseAlpha=off  SenseQDDot=off  SenseRDDot=off  SenseX=on  SenseY=on  SenseZ=on  SenseXYZ=off  SenseRad=off  SenseAzim=off  SenseDist=off  SenseInc=off  SenseXDot=off  SenseYDot=off  SenseZDot=off  SenseXYZDot=on  SenseRadDot=off  SenseAzimDot=off  SenseDistDot=off  SenseIncDot=off  SenseXDDot=off  SenseYDDot=off  SenseZDDot=off  SenseXYZDDot=off  SenseRadDDot=off  SenseAzimDDot=off  SenseDistDDot=off  SenseIncDDot=off
  Vector Concatenate : Concatenate  NumInputs=3
  World Frame : sm_lib/Frames and Transforms/World Frame
  Right Shoulder : PMIOPort  Side=Left
  Right Shoulder Torque : PMIOPort  Port=2  Side=Left
  Top of Right Arm : PMIOPort  Port=3  Side=Right
  RightShoulderVelocity : PMIOPort  Port=4  Side=Right
  RSonRArmFGlobalOut : Outport
  RSonRArmTGlobalOut : Outport  Port=2
  RS Global Position : Outport  Port=3
  wires:
  RotationMatrix/1 -> RSonRArmFGlob/1, RSonRArmTGlobal/1
  RSonRArmLocalForce/1 -> RSonRArmFGlob/2
  RSonRArmLocalTorque/1 -> RSonRArmTGlobal/2
  RSonRArmTGlobal/1 -> Dot Product2/1, RArmonRSTGlobal/1, RSonRArmTGlobalOut/1  "RSonRArmTGlobal"
  RSgx/1 -> Vector Concatenate/1
  RSgy/1 -> Vector Concatenate/2
  Vector Concatenate/1 -> RS Global Position/1  "RSGlobalPosition"
  RSgz/1 -> Vector Concatenate/3
  Dot Product1/1 -> RSLinearWorkonArm/1  "RSonArmLinearPower"
  Dot Product2/1 -> RSAngularWorkonArm/1  "RSonArmAngularPower"
  RSonRArmFGlob/1 -> RSLinearImpulseonArm/1, Dot Product1/1, RSonRArmFGlobalOut/1, RArmonRSFGlobal/1  "RSonRArmFGlobal"
  RSvGlobal/1 -> Dot Product1/2  "RSvGlobal"
  RSAV/1 -> Dot Product2/2  "RightShoulderGlobalAV"
  connections:
  Right Shoulder Torque/RConn1 -- Right Shoulder Revolute/LConn2
  Right Shoulder/RConn1 -- Right Shoulder Revolute/LConn1
  Spherical Solid/RConn1 -- Top of Right Arm/RConn1 -- Transform Sensor1/RConn1 -- Transform Sensor/RConn1 -- Right Shoulder Revolute/RConn1
  RSgx/LConn1 -- Transform Sensor/RConn3
  RotationMatrix/LConn1 -- Transform Sensor/RConn2
  RSgz/LConn1 -- Transform Sensor/RConn5
  RSgy/LConn1 -- Transform Sensor/RConn4
  World Frame/RConn1 -- Transform Sensor1/LConn1 -- Transform Sensor/LConn1
  Right Shoulder Revolute/RConn2 -- RightShoulderPosition/LConn1
  Right Shoulder Revolute/RConn4 -- RightShoulderAcceleration/LConn1
  Right Shoulder Revolute/RConn6 -- RSonRArmLocalTorque/LConn1 -- RightShoulderTorque/LConn1
  Right Shoulder Revolute/RConn3 -- RightShoulderVelocity/RConn1 -- RightShoulderVelocity1/LConn1
  Right Shoulder Revolute/RConn5 -- RSonRArmLocalForce/LConn1 -- RightShoulderForce/LConn1
  Transform Sensor1/RConn6 -- RSvGlobal/LConn1
  RSAV/LConn1 -- Transform Sensor1/RConn2
  Transform Sensor1/RConn5 -- RSz/LConn1
  Transform Sensor1/RConn4 -- RSy/LConn1
  Transform Sensor1/RConn3 -- RSx/LConn1
